simulink model "Position_Control_PID_CSEI"  (R2023b)
settings: Solver=FixedStepAuto  StartTime=0.0  StopTime=T_final  FixedStep=0.01  RelTol=1e-3
values from neighbouring files (symbols this model uses):
  current = [0;0]    [ASMC_ESO_sim_CSEI_Scripts.m]    (also in ASMC_FTESO_sim_CSEI_Scripts.m; Berthing_Control_PID_CSEI_Scripts.m; Position_Control_PID_CSEI_Scripts.m; Position_Control_PID_CSEI_Scripts_released.m)
  f_BT_max = 0.3*10    (= 3)    [Berthing_Control_PID_CSEI_Scripts.m]    (also in Control_allocation_test.m = 0.3; Position_Control_PID_CSEI_Scripts.m; Position_Control_PID_CSEI_Scripts_released.m; Waypoint_Control_PID_CSEI_Scripts.m)
  f_VSP1_max = 0.45*10    (= 4.5)    [Berthing_Control_PID_CSEI_Scripts.m]    (also in Control_allocation_test.m = 0.45; Position_Control_PID_CSEI_Scripts.m; Position_Control_PID_CSEI_Scripts_released.m; Waypoint_Control_PID_CSEI_Scripts.m)
  f_VSP2_max = 0.45*10    (= 4.5)    [Berthing_Control_PID_CSEI_Scripts.m]    (also in Control_allocation_test.m = 0.45; Position_Control_PID_CSEI_Scripts.m; Position_Control_PID_CSEI_Scripts_released.m; Waypoint_Control_PID_CSEI_Scripts.m)
  Fx_max = f_VSP1_max + f_VSP2_max    (= 9)    [Berthing_Control_PID_CSEI_Scripts.m]    (also in Control_allocation_test.m = 0.9; Position_Control_PID_CSEI_Scripts.m; Position_Control_PID_CSEI_Scripts_released.m; Waypoint_Control_PID_CSEI_Scripts.m)
  Fx_min = 0    [Berthing_Control_PID_CSEI_Scripts.m]    (also in Control_allocation_test.m = -0.9; Position_Control_PID_CSEI_Scripts.m; Position_Control_PID_CSEI_Scripts_released.m = -9; Waypoint_Control_PID_CSEI_Scripts.m)
  Fy_max = f_VSP1_max + f_VSP2_max + f_BT_max    (= 12)    [Berthing_Control_PID_CSEI_Scripts.m]    (also in Control_allocation_test.m = 1.2; Position_Control_PID_CSEI_Scripts.m; Position_Control_PID_CSEI_Scripts_released.m; Waypoint_Control_PID_CSEI_Scripts.m)
  Fy_min = -Fy_max    (= -12)    [Berthing_Control_PID_CSEI_Scripts.m]    (also in Control_allocation_test.m = -1.2; Position_Control_PID_CSEI_Scripts.m; Position_Control_PID_CSEI_Scripts_released.m; Waypoint_Control_PID_CSEI_Scripts.m)
  Kanti_u = 0.02    [Berthing_Control_PID_CSEI_Scripts.m]    (also in Position_Control_PID_CSEI_Scripts.m = 0; Waypoint_Control_PID_CSEI_Scripts.m; Waypoint_Control_PID_CSEI_Scripts_LLA.m)
  Kanti_x = 0    [Position_Control_PID_CSEI_Scripts.m]
  Kanti_y = 0    [Position_Control_PID_CSEI_Scripts.m]
  Kd_psi = 10    [Berthing_Control_PID_CSEI_Scripts.m]    (also in Position_Control_PID_CSEI_Scripts.m = 30; Waypoint_Control_PID_CSEI_Scripts.m; Waypoint_Control_PID_CSEI_Scripts_LLA.m)
  Kd_u = 1    [Berthing_Control_PID_CSEI_Scripts.m]    (also in Position_Control_PID_CSEI_Scripts.m = 7; Waypoint_Control_PID_CSEI_Scripts.m; Waypoint_Control_PID_CSEI_Scripts_LLA.m)
  Kd_v = 0    [Position_Control_PID_CSEI_Scripts.m]
  Kd_x = 0    [Position_Control_PID_CSEI_Scripts.m]
  Kd_y = 5    [Position_Control_PID_CSEI_Scripts.m]
  Ki_u = 2    [Berthing_Control_PID_CSEI_Scripts.m]    (also in Position_Control_PID_CSEI_Scripts.m = 0; Waypoint_Control_PID_CSEI_Scripts.m; Waypoint_Control_PID_CSEI_Scripts_LLA.m)
  Ki_x = 0    [Position_Control_PID_CSEI_Scripts.m]
  Ki_y = 0    [Position_Control_PID_CSEI_Scripts.m]
  Kp_psi = 100    [Berthing_Control_PID_CSEI_Scripts.m]    (also in Position_Control_PID_CSEI_Scripts.m = 50; Waypoint_Control_PID_CSEI_Scripts.m; Waypoint_Control_PID_CSEI_Scripts_LLA.m)
  Kp_u = 21    [Berthing_Control_PID_CSEI_Scripts.m]    (also in Position_Control_PID_CSEI_Scripts.m = 1; Waypoint_Control_PID_CSEI_Scripts.m; Waypoint_Control_PID_CSEI_Scripts_LLA.m)
  Kp_v = 1.2    [Position_Control_PID_CSEI_Scripts.m]
  Kp_x = 0.7    [Position_Control_PID_CSEI_Scripts.m]
  Kp_y = 0.3    [Position_Control_PID_CSEI_Scripts.m]
  N_max = Fx_max*ly_VSP*(1) - Fx_max*ly_VSP*(-1) + f_BT_max*lx_BT    (= 2.1525)    [Berthing_Control_PID_CSEI_Scripts.m]    (also in Control_allocation_test.m = 0.16575; Position_Control_PID_CSEI_Scripts.m; Position_Control_PID_CSEI_Scripts_released.m; Waypoint_Control_PID_CSEI_Scripts.m)
  N_min = -N_max    (= -2.1525)    [Berthing_Control_PID_CSEI_Scripts.m]    (also in Control_allocation_test.m = -0.16575; Position_Control_PID_CSEI_Scripts.m; Position_Control_PID_CSEI_Scripts_released.m; Waypoint_Control_PID_CSEI_Scripts.m)
  Nu = 100    [Position_Control_PID_CSEI_Scripts.m]
  Nv = 100    [Position_Control_PID_CSEI_Scripts.m]
  Nx = 100    [Position_Control_PID_CSEI_Scripts.m]
  Ny = 100    [Position_Control_PID_CSEI_Scripts.m]
  psi_ref_deg = 50    [Position_Control_PID_CSEI_Scripts.m]    (also in Position_Control_PID_CSEI_Scripts_released.m = 30)
  u_max = 2    [Position_Control_PID_CSEI_Scripts.m]    (also in Position_Control_PID_CSEI_Scripts_released.m)
  u_min = -2    [Position_Control_PID_CSEI_Scripts.m]    (also in Position_Control_PID_CSEI_Scripts_released.m)
  u_vsp_min = 0    [Position_Control_PID_CSEI_Scripts.m]    (also in Position_Control_PID_CSEI_Scripts_released.m)
  v_max = 10    [ASMC_ESO_sim_CSEI_Scripts.m]    (also in ASMC_FTESO_sim_CSEI_Scripts.m; Position_Control_PID_CSEI_Scripts.m = 2; Position_Control_PID_CSEI_Scripts_released.m = 2; SMC_ESO_sim_CSEI_Scripts.m)
  v_min = -v_max    (= -0.25)    [ASMC_ESO_sim_CSEI_Scripts.m]    (also in ASMC_FTESO_sim_CSEI_Scripts.m; Position_Control_PID_CSEI_Scripts.m = -2; Position_Control_PID_CSEI_Scripts_released.m = -2; SMC_ESO_sim_CSEI_Scripts.m)
  x0 = zeros(6,1)    [Berthing_Control_PID_CSEI_Scripts.m]    (also in Position_Control_PID_CSEI_Scripts.m; Position_Control_PID_CSEI_Scripts_released.m; Waypoint_Control_PID_CSEI_Scripts.m; Waypoint_Control_PID_CSEI_Scripts_LLA.m)
  x_dock = 20    [Position_Control_PID_CSEI_Scripts.m]    (also in Position_Control_PID_CSEI_Scripts_released.m = 30)
  y_dock = 20    [Position_Control_PID_CSEI_Scripts.m]    (also in Position_Control_PID_CSEI_Scripts_released.m = 30)
libraries: simulink_extras x4, vrlib x2
settings Model: Creator=ADMIN  LastModifiedBy=ADMIN
settings ModelReferenceCC: EnableRefExpFcnMdlSchedulingChecks=on

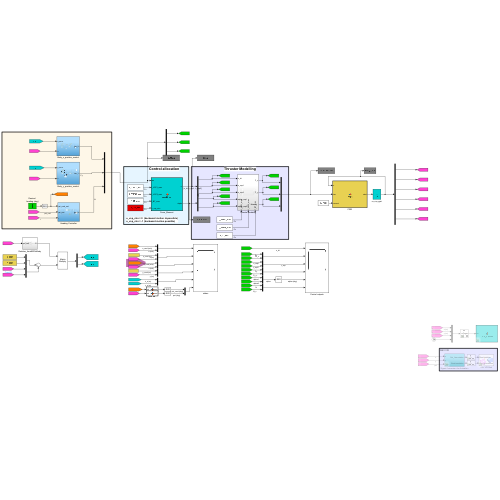
[thumbnail: Simulink's stored preview of the top-level diagram]
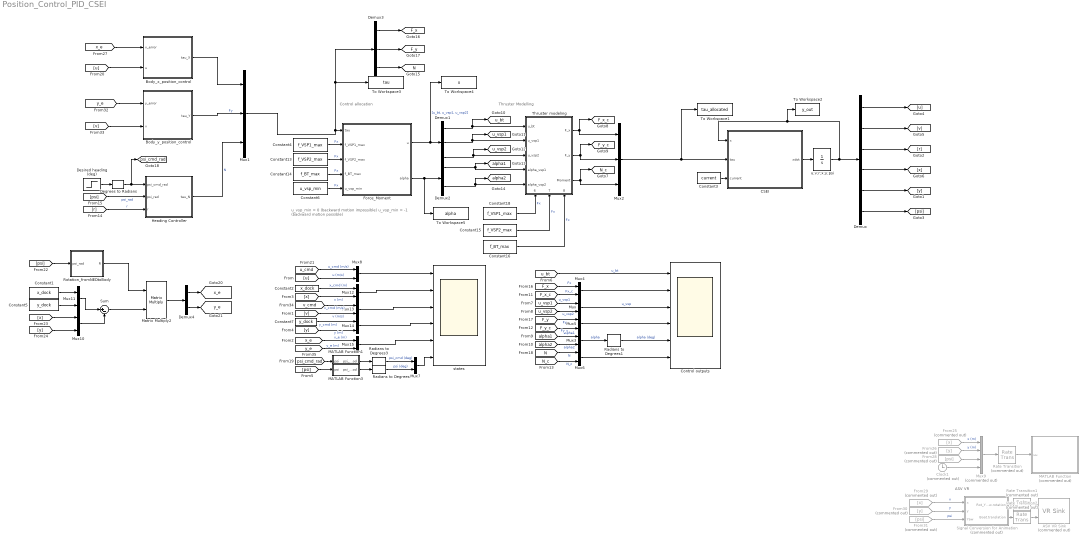
== system Position_Control_PID_CSEI ==
  note: u_vsp_min = 0 (backward motion impossible)
      | u_vsp_min = -1 (backward motion possible)
  note: Thruster Modelling
  note: ASV VR
  note: Control allocation
  ASV VR Sink : vrlib/VR Sink  Commented=on  InstantiateOnLoad=on  SampleTime=0.1  ViewEnable=on  RemoteChange=off  RemoteView=off  FieldsWritten=Boat.rotation.4.1.1.double#Boat.translation.3.1.1.double  WorldFileName=ASV.x3d  WorldDescription=ASV Simulation Animation  AutoView=off  VideoDimensions=[]  AllowVariableSize=off
  Body_x_position_control : Subsystem
  Body_y_position_control : Subsystem
  CSEI : MATLAB Function  TreatAsAtomicUnit=on
  Clock1 : Clock  Commented=on
  Constant1 : Constant  Value=x_dock
  Constant13 : Constant  Value=f_VSP2_max
  Constant14 : Constant  Value=f_BT_max
  Constant15 : Constant  Value=f_VSP2_max
  Constant16 : Constant  Value=f_BT_max
  Constant18 : Constant  Value=f_VSP1_max
  Constant2 : Constant  Value=x_dock
  Constant3 : Constant  Value=current
  Constant4 : Constant  Value=f_VSP1_max
  Constant5 : Constant  Value=y_dock
  Constant6 : Constant  Value=u_vsp_min
  Constant7 : Constant  Value=y_dock
  Control outputs : Scope  NumInputPorts=6
  Degrees to Radians : simulink_extras/Transformations/Degrees to Radians
  Demux : Demux  Outputs=6
  Demux1 : Demux  Outputs=3
  Demux2 : Demux  Outputs=2
  Demux3 : Demux  Outputs=3
  Demux4 : Demux  Outputs=2
  Desired heading (deg) : Step  Time=0  After=psi_ref_deg  SampleTime=0
  Force_Moment : MATLAB Function  TreatAsAtomicUnit=on
  From25 : From  Commented=on  GotoTag=x
  From26 : From  Commented=on  GotoTag=y
  From28 : From  Commented=on  GotoTag=psi
  From29 : From  Commented=on  GotoTag=x
  From30 : From  Commented=on  GotoTag=y
  From31 : From  Commented=on  GotoTag=psi
  Heading Controller : Subsystem
  MATLAB Function : MATLAB Function  Commented=on  TreatAsAtomicUnit=on
  MATLAB Function1 : MATLAB Function  TreatAsAtomicUnit=on
  MATLAB Function3 : MATLAB Function  TreatAsAtomicUnit=on
  Matrix Multiply2 : Product  Multiplication=Matrix(*)
  Mux{,3..8,10..15} (13 alike) : Mux  Inputs=2
  Mux1 : Mux  Inputs=3
  Mux2 : Mux  Inputs=3
  Mux9 : Mux  Commented=on
  Radians to Degrees : simulink_extras/Transformations/Radians to Degrees
  Radians to Degrees1 : simulink_extras/Transformations/Radians to Degrees
  Radians to Degrees3 : simulink_extras/Transformations/Radians to Degrees
  Rate Transition : RateTransition  Commented=on  OutPortSampleTime=5
  Rate Transition1 : RateTransition  Commented=on  OutPortSampleTime=5
  Rate Transition2 : RateTransition  Commented=on  OutPortSampleTime=5
  Rotation_fromNEDtoBody : Subsystem
  Signal Conversion for Animation : Subsystem  Commented=on
  Sum : Sum  Inputs=|+-
  Thruster modeling : Subsystem
      settings: PortSchema="{\"entries\":[{\"content\":{\"sides\":[{\"content\":{\"connectorIds\":[\"In1\",\"In2\",\"In3\",\"In4\",\"In5\"]},\"type\":\"ConnectorPlacement.EquallySpacedRectSide\",\"uuid\":\"a022356d-9f83-420f-8db1-af87d581b43a\"},{\"content\":{\"connectorIds\":[\"Out1\",\"Out2\",\"Out3\"],\"side\":\"RIGHT\"},\"type\":\"ConnectorPlacement.EquallySpacedRectSide\",\"uuid\":\"80059f0e-998a-4ca1-ad21-b5517d0d415e\"},{\"content\":{\"side\":\"TOP\"},\"type\":\"ConnectorPlacement.EquallySpacedRectSide\",\"uuid\":\"bbd861b1-62fd-403d-9398-039fcb3ecf9c\"},{\"content\":{\"connectorIds\":[\"In6\",\"In7\",\"In8\"],\"side\":\"BOTTOM\"},\"type\":\"ConnectorPlacement.EquallySpacedRectSide\",\"uuid\":\"ab01237b-8b46-48b2-b107-c489b1f78e8c\"}]},\"type\":\"ConnectorPlacement.EquallySpacedConnector\",\"uuid\":\"7da2a0ce-fa7c-4136-9950-942e5a1638e8\"}],\"packageUris\":[\"http://schema.mathworks.com/mf0/Connector/R2020b\"],\"version\":\"1.0\"}"
  To Workspace1 : ToWorkspace  VariableName=tau_allocated  SampleTime=-1
  To Workspace2 : ToWorkspace  VariableName=y_out  SampleTime=-1
  To Workspace3 : ToWorkspace  VariableName=tau  SampleTime=-1
  To Workspace4 : ToWorkspace  VariableName=u  SampleTime=-1
  To Workspace5 : ToWorkspace  VariableName=alpha  SampleTime=-1
  states : Scope  NumInputPorts=6
  u;v;r;x;y;psi : Integrator  InitialCondition=x0
  tag scope: F_x=global, F_x_c=global, F_y=global, F_y_c=global, N=global, N_c=global, alpha1=global, alpha2=global, psi_cmd_rad=global, u_bt=global, u_vsp1=global, u_vsp2=global, x_e=global, y_e=global
  wires:
  Mux2/1 -> To Workspace1/1, CSEI/2(tau)
  CSEI/1(xdot) -> u;v;r;x;y;psi/1
  u;v;r;x;y;psi/1 -> Demux/1, To Workspace2/1, CSEI/1(x)
  Constant3/1 -> CSEI/3(current)
  Thruster modeling/1(F_x) -> Mux2/1, [F_x_c]
  Thruster modeling/2(F_y) -> Mux2/2, [F_y_c]
  Thruster modeling/3("Moment ") -> Mux2/3, [N_c]
  Demux/6 -> [psi]
  Demux/1 -> [u]
  Demux/4 -> [x]
  Demux/5 -> [y]
  Demux/3 -> [r]
  Demux/2 -> [v]
  Demux2/1 -> Thruster modeling/4(alpha_vsp1), [alpha1]
  Demux1/2 -> Thruster modeling/2(u_vsp1), [u_vsp1]
  Demux1/1 -> Thruster modeling/1(u_bt), [u_bt]
  [u_vsp1] -> Mux/1  "u_vsp1"
  [u_vsp2] -> Mux/2  "u_vsp2"
  [alpha1] -> Mux3/1  "alpha1"
  [alpha2] -> Mux3/2  "alpha2"
  [u_bt] -> Control outputs/1  "u_bt"
  Mux/1 -> Control outputs/3  "u_vsp"
  [F_x_c] -> Mux4/2  "Fx_c"
  Mux3/1 -> Radians to Degrees1/1  "alpha"
  Radians to Degrees1/1 -> Control outputs/5  "alpha (deg)"
  Demux2/2 -> [alpha2], Thruster modeling/5(alpha_vsp2)
  Demux1/3 -> [u_vsp2], Thruster modeling/3("u_vsp2 ")
  Force_Moment/1(u) -> To Workspace4/1, Demux1/1  "[u_bt, u_vsp1, u_vsp2]"
  Force_Moment/2(alpha) -> To Workspace5/1, Demux2/1
  [psi] -> Heading Controller/2(psi_rad)  "psi_rad"
  [r] -> Heading Controller/3(r)  "r"
  Heading Controller/1(tau_N) -> Mux1/3  "N"
  Body_y_position_control/1(tau_Y) -> Mux1/2  "Fy"
  [F_x] -> Mux4/1  "Fx"
  Mux4/1 -> Control outputs/2
  [F_y] -> Mux5/1  "Fy"
  [F_y_c] -> Mux5/2  "Fy_c"
  Mux5/1 -> Control outputs/4
  [N] -> Mux6/1  "N"
  [N_c] -> Mux6/2  "N_c"
  Mux6/1 -> Control outputs/6
  Constant4/1 -> Force_Moment/2(f_VSP1_max)  "Fx"
  [u] -> Body_x_position_control/2(u)
  Body_x_position_control/1(tau_X) -> Mux1/1
  Clock1/1 -> Mux9/4
  From26/1 -> Mux9/2  "y (m)"
  From25/1 -> Mux9/1  "x (m)"
  Mux9/1 -> Rate Transition/1
  From28/1 -> Mux9/3
  Rate Transition/1 -> MATLAB Function/1(uu)
  Signal Conversion for Animation/1(Rot_Yaw.rotation) -> Rate Transition1/1
  Signal Conversion for Animation/2(Boat.translation) -> Rate Transition2/1
  From30/1 -> Signal Conversion for Animation/2(y)  "y"
  From31/1 -> Signal Conversion for Animation/3(Yaw)  "psi"
  From29/1 -> Signal Conversion for Animation/1(x)  "x"
  Rate Transition1/1 -> ASV VR Sink/1
  Rate Transition2/1 -> ASV VR Sink/2
  Degrees to Radians/1 -> [psi_cmd_rad], Heading Controller/1(psi_cmd_rad)
  Mux1/1 -> Demux3/1, To Workspace3/1, Force_Moment/1(tau)
  Demux3/1 -> [F_x]
  Demux3/2 -> [F_y]
  Demux3/3 -> [N]
  Constant13/1 -> Force_Moment/3(f_VSP2_max)  "Fx"
  Constant14/1 -> Force_Moment/4(f_BT_max)  "Fx"
  Constant18/1 -> Thruster modeling/6(f_VSP1_max)  "Fx"
  Constant15/1 -> Thruster modeling/7(f_VSP2_max)  "Fx"
  Constant16/1 -> Thruster modeling/8(f_BT_max)  "Fx"
  Desired heading (deg)/1 -> Degrees to Radians/1
  [psi] -> Rotation_fromNEDtoBody/1(psi_rad)
  Demux4/2 -> [y_e]
  Rotation_fromNEDtoBody/1(R) -> Matrix Multiply2/1
  Matrix Multiply2/1 -> Demux4/1
  Demux4/1 -> [x_e]
  [x] -> Mux10/1
  Sum/1 -> Matrix Multiply2/2
  [y] -> Mux10/2
  Constant5/1 -> Mux11/2
  Constant1/1 -> Mux11/1
  Mux11/1 -> Sum/1
  Mux10/1 -> Sum/2
  [x_e] -> Body_x_position_control/1(x_error)
  [y_e] -> Body_y_position_control/1(y_error)
  [v] -> Body_y_position_control/2(v)
  Constant2/1 -> Mux12/1  "x_cmd (m)"
  Radians to Degrees3/1 -> Mux7/1  "psi_cmd (deg)"
  [v] -> Mux13/2  "v (m/s)"
  [psi_cmd_rad] -> MATLAB Function1/1(psi)
  Mux8/1 -> states/1
  Mux15/1 -> states/5
  [u_cmd] -> Mux8/1  "u_cmd (m/s)"
  Mux7/1 -> states/6
  MATLAB Function1/1(psi_mod) -> Radians to Degrees3/1
  [psi] -> MATLAB Function3/1(psi)
  [x] -> Mux12/2  "x (m)"
  [y] -> Mux14/2  "y (m)"
  Mux12/1 -> states/2
  Radians to Degrees/1 -> Mux7/2  "psi (deg)"
  MATLAB Function3/1(psi_mod) -> Radians to Degrees/1
  [u] -> Mux8/2  "u (m/s)"
  Mux13/1 -> states/3
  [v_cmd] -> Mux13/1  "v_cmd (m/s)"
  Mux14/1 -> states/4
  Constant7/1 -> Mux14/1  "y_cmd (m)"
  [x_e] -> Mux15/1  "x_e (m)"
  [y_e] -> Mux15/2  "y_e (m)"
  Constant6/1 -> Force_Moment/5(u_vsp_min)  "Fx"

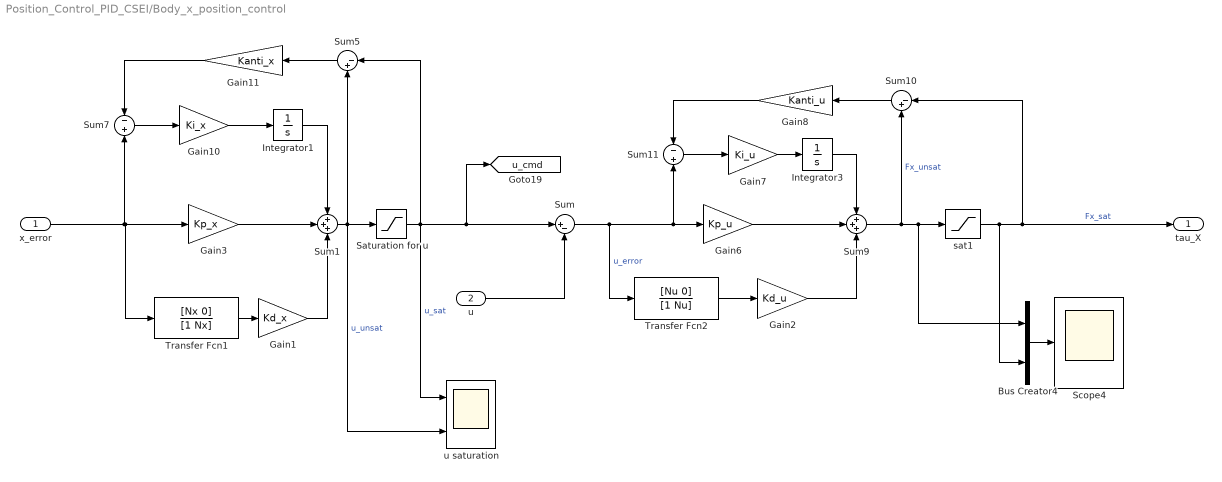
== system Position_Control_PID_CSEI/Body_x_position_control ==
  x_error : Inport
  u : Inport  Port=2
  Bus Creator4 : BusCreator  Inputs=2
  Gain1 : Gain  Gain=Kd_x
  Gain10 : Gain  Gain=Ki_x
  Gain11 : Gain  Gain=Kanti_x
  Gain2 : Gain  Gain=Kd_u
  Gain3 : Gain  Gain=Kp_x
  Gain6 : Gain  Gain=Kp_u
  Gain7 : Gain  Gain=Ki_u
  Gain8 : Gain  Gain=Kanti_u
  Integrator1 : Integrator
  Integrator3 : Integrator
  Saturation for u : Saturate  UpperLimit=u_max  LowerLimit=u_min
  Scope4 : Scope
  Sum : Sum  Inputs=|+-
  Sum1 : Sum  Inputs=+++  InputSameDT=on  SaturateOnIntegerOverflow=on  OutDataTypeStr=Inherit: Same as first input
  Sum10 : Sum  Inputs=|-+  InputSameDT=on  SaturateOnIntegerOverflow=on  OutDataTypeStr=Inherit: Same as first input
  Sum11 : Sum  Inputs=-|+  InputSameDT=on  SaturateOnIntegerOverflow=on  OutDataTypeStr=Inherit: Same as first input
  Sum5 : Sum  Inputs=|-+  InputSameDT=on  SaturateOnIntegerOverflow=on  OutDataTypeStr=Inherit: Same as first input
  Sum7 : Sum  Inputs=-|+  InputSameDT=on  SaturateOnIntegerOverflow=on  OutDataTypeStr=Inherit: Same as first input
  Sum9 : Sum  Inputs=+++  InputSameDT=on  SaturateOnIntegerOverflow=on  OutDataTypeStr=Inherit: Same as first input
  Transfer Fcn1 : TransferFcn  Numerator=[Nx 0]  Denominator=[1 Nx]
  Transfer Fcn2 : TransferFcn  Numerator=[Nu 0]  Denominator=[1 Nu]
  sat1 : Saturate  UpperLimit=Fx_max  LowerLimit=Fx_min
      settings: AttributesFormatString=%<LowerLimit>~%<UpperLimit>
  u saturation : Scope  NumInputPorts=2
  tau_X : Outport
  tag scope: u_cmd=global
  wires:
  Gain7/1 -> Integrator3/1
  Sum/1 -> Transfer Fcn2/1, Gain6/1, Sum11/2  "u_error"
  sat1/1 -> tau_X/1, Sum10/1, Bus Creator4/2  "Fx_sat"
  Bus Creator4/1 -> Scope4/1
  Transfer Fcn2/1 -> Gain2/1
  Sum9/1 -> Bus Creator4/1, sat1/1, Sum10/2  "Fx_unsat"
  Sum10/1 -> Gain8/1
  Integrator3/1 -> Sum9/1
  Gain2/1 -> Sum9/3
  Gain8/1 -> Sum11/1
  Gain6/1 -> Sum9/2
  Sum11/1 -> Gain7/1
  u/1 -> Sum/2
  Sum5/1 -> Gain11/1
  Saturation for u/1 -> [u_cmd], Sum/1, u saturation/1, Sum5/1  "u_sat"
  Sum7/1 -> Gain10/1
  Gain3/1 -> Sum1/2
  Gain11/1 -> Sum7/1
  Integrator1/1 -> Sum1/1
  Gain1/1 -> Sum1/3
  Sum1/1 -> u saturation/2, Sum5/2, Saturation for u/1  "u_unsat"
  Gain10/1 -> Integrator1/1
  x_error/1 -> Transfer Fcn1/1, Gain3/1, Sum7/2
  Transfer Fcn1/1 -> Gain1/1

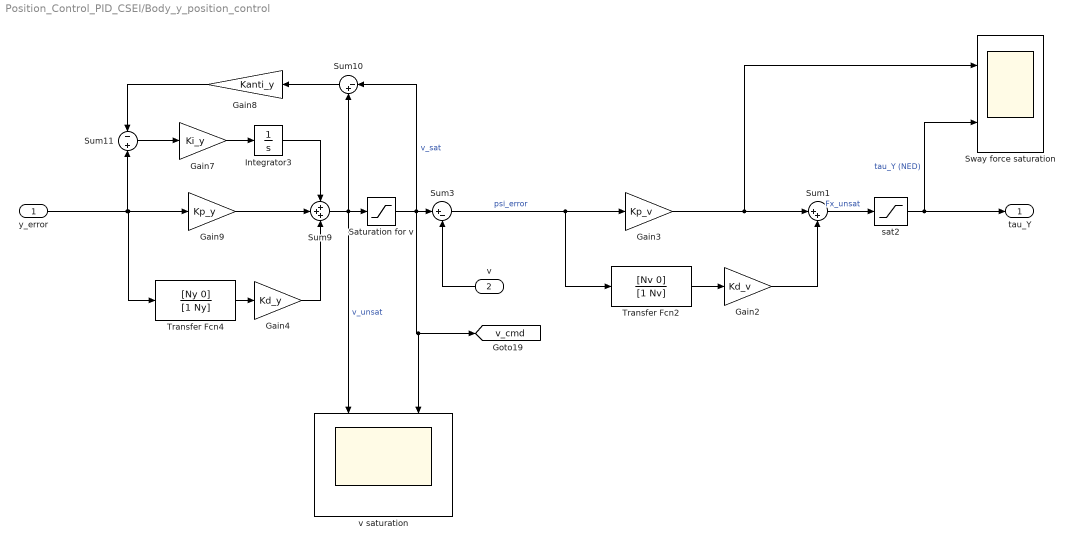
== system Position_Control_PID_CSEI/Body_y_position_control ==
  y_error : Inport
  v : Inport  Port=2
  Gain2 : Gain  Gain=Kd_v
  Gain3 : Gain  Gain=Kp_v
  Gain4 : Gain  Gain=Kd_y
  Gain7 : Gain  Gain=Ki_y
  Gain8 : Gain  Gain=Kanti_y
  Gain9 : Gain  Gain=Kp_y
  Integrator3 : Integrator
  Saturation for v : Saturate  UpperLimit=v_max  LowerLimit=v_min
  Sum1 : Sum  Inputs=|++  InputSameDT=on  SaturateOnIntegerOverflow=on  OutDataTypeStr=Inherit: Same as first input
  Sum10 : Sum  Inputs=|-+  InputSameDT=on  SaturateOnIntegerOverflow=on  OutDataTypeStr=Inherit: Same as first input
  Sum11 : Sum  Inputs=-|+  InputSameDT=on  SaturateOnIntegerOverflow=on  OutDataTypeStr=Inherit: Same as first input
  Sum3 : Sum  Inputs=|+-  InputSameDT=on  SaturateOnIntegerOverflow=on  OutDataTypeStr=Inherit: Same as first input
  Sum9 : Sum  Inputs=+++  InputSameDT=on  SaturateOnIntegerOverflow=on  OutDataTypeStr=Inherit: Same as first input
  Sway force saturation : Scope  NumInputPorts=2
  Transfer Fcn2 : TransferFcn  Numerator=[Nv 0]  Denominator=[1 Nv]
  Transfer Fcn4 : TransferFcn  Numerator=[Ny 0]  Denominator=[1 Ny]
  sat2 : Saturate  UpperLimit=Fy_max  LowerLimit=Fy_min
      settings: AttributesFormatString=%<LowerLimit>~%<UpperLimit>
  v saturation : Scope  NumInputPorts=2
  tau_Y : Outport
  tag scope: v_cmd=global
  wires:
  Sum10/1 -> Gain8/1
  y_error/1 -> Sum11/2, Gain9/1, Transfer Fcn4/1
  Gain3/1 -> Sum1/1, Sway force saturation/1
  sat2/1 -> Sway force saturation/2, tau_Y/1  "tau_Y (NED)"
  Gain9/1 -> Sum9/2
  Saturation for v/1 -> [v_cmd], v saturation/2, Sum10/1, Sum3/1  "v_sat"
  Gain7/1 -> Integrator3/1
  Sum11/1 -> Gain7/1
  Integrator3/1 -> Sum9/1
  Gain8/1 -> Sum11/1
  Sum9/1 -> v saturation/1, Sum10/2, Saturation for v/1  "v_unsat"
  Transfer Fcn4/1 -> Gain4/1
  Gain4/1 -> Sum9/3
  Sum3/1 -> Transfer Fcn2/1, Gain3/1  "psi_error"
  v/1 -> Sum3/2
  Transfer Fcn2/1 -> Gain2/1
  Gain2/1 -> Sum1/2
  Sum1/1 -> sat2/1  "Fx_unsat"

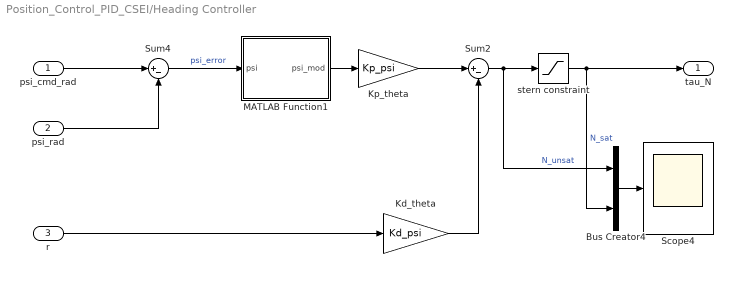
== system Position_Control_PID_CSEI/Heading Controller ==
  psi_cmd_rad : Inport
  psi_rad : Inport  Port=2
  r : Inport  Port=3
  Bus Creator4 : BusCreator  Inputs=2
  Kd_theta : Gain  Gain=Kd_psi  SaturateOnIntegerOverflow=on  OutDataTypeStr=Inherit: Same as input  ParamDataTypeStr=Inherit: Same as input
  Kp_theta : Gain  Gain=Kp_psi  SaturateOnIntegerOverflow=on  OutDataTypeStr=Inherit: Same as input  ParamDataTypeStr=Inherit: Same as input
  MATLAB Function1 : MATLAB Function  TreatAsAtomicUnit=on
  Scope4 : Scope
  Sum2 : Sum  Inputs=|+-  InputSameDT=on  SaturateOnIntegerOverflow=on  OutDataTypeStr=Inherit: Same as first input
  Sum4 : Sum  Inputs=|+-  InputSameDT=on  SaturateOnIntegerOverflow=on  OutDataTypeStr=Inherit: Same as first input
  stern constraint : Saturate  UpperLimit=N_max  LowerLimit=N_min
      settings: AttributesFormatString=%<LowerLimit>~%<UpperLimit>
  tau_N : Outport
  wires:
  Kp_theta/1 -> Sum2/1
  MATLAB Function1/1(psi_mod) -> Kp_theta/1
  psi_cmd_rad/1 -> Sum4/1
  Sum4/1 -> MATLAB Function1/1(psi)  "psi_error"
  Kd_theta/1 -> Sum2/2
  r/1 -> Kd_theta/1
  psi_rad/1 -> Sum4/2
  Sum2/1 -> Bus Creator4/1, stern constraint/1  "N_unsat"
  Bus Creator4/1 -> Scope4/1
  stern constraint/1 -> Bus Creator4/2, tau_N/1  "N_sat"

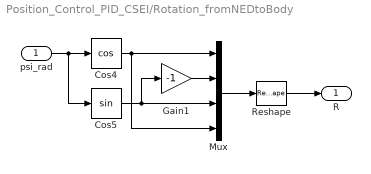
== system Position_Control_PID_CSEI/Rotation_fromNEDtoBody ==
  psi_rad : Inport
  Cos4 : Trigonometry  Operator=cos
  Cos5 : Trigonometry
  Gain1 : Gain  Gain=-1
  Mux : Mux
  Reshape : Reshape  OutputDimensionality=Customize  OutputDimensions=[2,2]
  R : Outport
  wires:
  psi_rad/1 -> Cos5/1, Cos4/1
  Mux/1 -> Reshape/1
  Cos4/1 -> Mux/1, Mux/4
  Cos5/1 -> Mux/3, Gain1/1
  Reshape/1 -> R/1
  Gain1/1 -> Mux/2

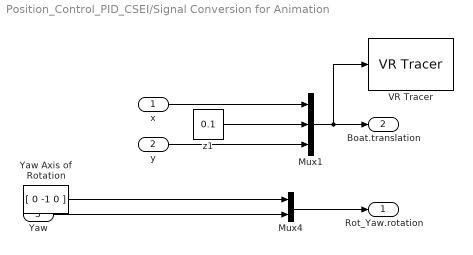
== system Position_Control_PID_CSEI/Signal Conversion for Animation ==
  x : Inport
  y : Inport  Port=2
  Yaw : Inport  Port=3
  Mux1 : Mux  Inputs=3
  Mux4 : Mux  Inputs=2
  VR Tracer : vrlib/VR Tracer  VrmlFile=ASV.x3d  MarkerName=None  UseLines=on  UseTriads=off  MarkerScale=[1 1 1]  MarkerColorSelection=Defined as RGB values  MarkerColor=red  rgbval=[1 0 0]  Ts=0.5  ForceViewerOpen=off  ConnectPlane=off  PlaneCoeff=[0 1 0 0]  ConnectPoint=None  PointCoord=[0 0 0]
  Yaw Axis of Rotation : Constant  Value=[ 0 -1 0 ]
  z1 : Constant  Value=0.1
  Rot_Yaw.rotation : Outport
  Boat.translation : Outport  Port=2
  wires:
  Yaw Axis of Rotation/1 -> Mux4/1
  Mux1/1 -> VR Tracer/1, Boat.translation/1
  x/1 -> Mux1/1
  Mux4/1 -> Rot_Yaw.rotation/1
  Yaw/1 -> Mux4/2
  y/1 -> Mux1/3
  z1/1 -> Mux1/2

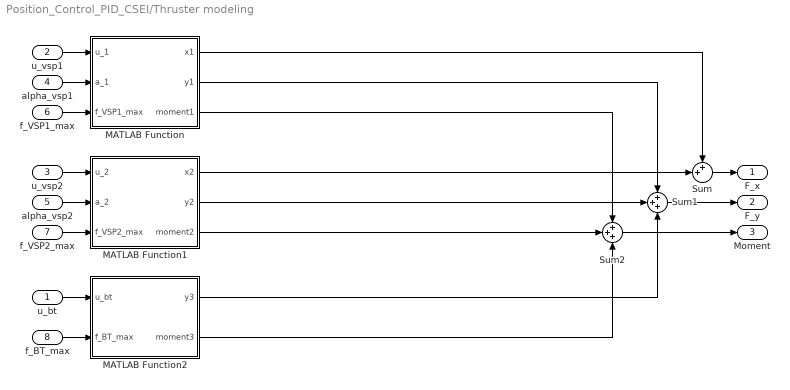
== system Position_Control_PID_CSEI/Thruster modeling ==
  u_bt : Inport
  u_vsp1 : Inport  Port=2
  "u_vsp2 " : Inport  Port=3
  alpha_vsp1 : Inport  Port=4
  alpha_vsp2 : Inport  Port=5
  f_VSP1_max : Inport  Port=6
  f_VSP2_max : Inport  Port=7
  f_BT_max : Inport  Port=8
  MATLAB Function : MATLAB Function  TreatAsAtomicUnit=on
  MATLAB Function1 : MATLAB Function  TreatAsAtomicUnit=on
  MATLAB Function2 : MATLAB Function  TreatAsAtomicUnit=on
  Sum : Sum  Inputs=++|
  Sum1 : Sum  Inputs=+++
  Sum2 : Sum  Inputs=+++
  F_x : Outport
  F_y : Outport  Port=2
  "Moment " : Outport  Port=3
  wires:
  u_bt/1 -> MATLAB Function2/1(u_bt)
  alpha_vsp2/1 -> MATLAB Function1/2(a_2)
  u_vsp1/1 -> MATLAB Function/1(u_1)
  "u_vsp2 "/1 -> MATLAB Function1/1(u_2)
  MATLAB Function1/1(x2) -> Sum/2
  Sum/1 -> F_x/1
  Sum1/1 -> F_y/1
  MATLAB Function1/2(y2) -> Sum1/2
  MATLAB Function2/1(y3) -> Sum1/3
  Sum2/1 -> "Moment "/1
  MATLAB Function2/2(moment3) -> Sum2/3
  MATLAB Function1/3(moment2) -> Sum2/2
  MATLAB Function/3(moment1) -> Sum2/1
  MATLAB Function/1(x1) -> Sum/1
  MATLAB Function/2(y1) -> Sum1/1
  alpha_vsp1/1 -> MATLAB Function/2(a_1)
  f_VSP1_max/1 -> MATLAB Function/3(f_VSP1_max)
  f_VSP2_max/1 -> MATLAB Function1/3(f_VSP2_max)
  f_BT_max/1 -> MATLAB Function2/2(f_BT_max)

== matlab function Position_Control_PID_CSEI/Force_Moment ==
  data: tau input; u output; alpha output; f_VSP1_max input; f_VSP2_max input; f_BT_max input; u_vsp_min input
function [u, alpha] = force2input(tau, f_VSP1_max, f_VSP2_max, f_BT_max, u_vsp_min)
    % Mapping of desired force (tau) to input to the actuators (u)
    % Input: 3DOF desired forces and moment in body-frame, tau = [X Y N]'
    % Output: input signals to the actuators, u = [u_BT u_VSP1 u_VSP2]';
    %         angles of the two VSPs, alpha = [alpha_VSP1 alpha_VSP2]';
    %         angular rates of the VSPs, omega = [omega_VSP1 omega_VSP2]'
%% Initializing values
    ly_VSP = 0.055;         % Moment arm along y for VSP
    lx_VSP = 0.4574;        % Moment arm along x for VSP
    lx_BT = 0.3875;         % Moment arm along x for BT

    % test
    alpha = zeros(2,1);     % VSP angles
    u = zeros(3,1);         % Input vector to the VSPs and BT

    B = [  1      0       1      0      0;
           0      1       0      1      1;
         ly_VSP -lx_VSP -ly_VSP -lx_VSP lx_BT]; % Configuration matrix
%% Thrust allocation
    B_inv = pinv(B);                         % Calculating dagger
    f_cmd = B_inv*tau;                       % Forces and moment

    u_cmd = [norm(f_cmd(1:2))/f_VSP1_max;
             norm(f_cmd(3:4))/f_VSP2_max;
             f_cmd(5)/f_BT_max];                % Calculating input to each
                                                % thruster
    % Saturation: Limit input signal to VSPs to be within [0,1]
    if u_cmd(1) < u_vsp_min
        u_cmd(1) = u_vsp_min;
    elseif u_cmd(1) > 1
        u_cmd(1) = 1;
    else
        u_cmd(1) = u_cmd(1);
    end

    if u_cmd(2) < u_vsp_min
        u_cmd(2) = u_vsp_min;
    elseif u_cmd(2) > 1
        u_cmd(2) = 1;
    else
        u_cmd(2) = u_cmd(2);
    end

    % Saturation: Limit input signal to BT to be within [-1,1]
    if u_cmd(3) < -1
        u_cmd(3) = -1;
    elseif u_cmd(3) > 1
        u_cmd(3) = 1;
    else
        u_cmd(3) = u_cmd(3);
    end
    
    alpha(1) = atan2(f_cmd(2),f_cmd(1));         % Calculate angle of VSP1
    alpha(2) = atan2(f_cmd(4),f_cmd(3));         % Calculate angle of VSP2
    BT_gain = 1;                                 % Gain used in LAB

    u(1) = u_cmd(3)*BT_gain;                     % Output input to BT
    u(2) = u_cmd(1);                             % Output input to VSP1
    u(3) = u_cmd(2);                             % Output input to VSP2
    
end

== matlab function Position_Control_PID_CSEI/Heading Controller/MATLAB Function1 ==
  data: psi input; psi_mod output
function psi_mod = wrapToPi(psi)

psi_mod = mod(psi + pi, 2*pi) - pi;

== matlab function Position_Control_PID_CSEI/MATLAB Function3 ==
  data: psi input; psi_mod output
function psi_mod = wrapToPi(psi)

psi_mod = mod(psi + pi, 2*pi) - pi;

== matlab function Position_Control_PID_CSEI/CSEI ==
  data: xdot output; x input; tau input; current input
function xdot  = CSEI(x, tau, current)
%% nu = [u, v, r], eta = [x, y, psi]
%  u:     surge velocity          (m/s)
%  v:     sway velocity           (m/s)
%  r:     yaw velocity            (rad/s)
%  x:     position in x direction (m)
%  y:     position in y direction (m)
%  psi:   yaw angle               (rad)

% This block calculates the change in position and heading given the
% current position and heading and velocities.


% State and current variables
nu = x(1:3); eta = x(4:6);
%% Initializing parameters
R = [cos(eta(3)) -sin(eta(3)) 0;
     sin(eta(3)) cos(eta(3)) 0;
     0 0 1];                        % Rotation matrix with heading
nu_c = R'*[current;0];              % Current velocity vector in body frame
nu_r = nu-nu_c;                     % Relative velocity
u   = nu_r(1);                      % Speed in x
v   = nu_r(2);                      % Speed in y
r   = nu_r(3);                      % Yaw rate

tau = [tau(1);tau(2);tau(3)];
%% MATRICES 
m    = 14.11;   I_z  =  1.7600;   x_g = 0.0375;

%% Added mass
X_ud  =     -2.0;											
					Y_vd =      -10.0;	N_vd =    -0.0;		
					Y_rd =      -0.0;	N_rd =    -1.0;	

%% Total mass matrix
m_11 = m-X_ud;
m_22 = m-Y_vd;
m_23 = m*x_g-Y_rd;
m_32 = m*x_g-N_vd;
m_33 = I_z-N_rd;

M    = [m_11 0    0
        0    m_22 m_23
        0    m_32 m_33];
	
%% Damping coefficients
% Comments at the end of the lines indicate the old values used.
X_u		= -0.6555;		X_v		= 0;
X_uu 	= 0.3545;		X_vv	= -2.443;
X_uuu 	= -3.787;		X_vvv	= 0;

						Y_v		= -1.33; 			Y_r		= -7.250; 
						Y_vv	= -2.776;			Y_rr	= -3.450; 
						Y_vvv	= -64.91;			Y_rrr	= 0;
						
						Y_rv	= -0.805;			Y_vr	= -0.845;

						N_v		= 0;				N_r		= -1.900;
						N_vv	= -0.2088;			N_rr	= -0.750;
						N_vvv	= 0;				N_rrr	= 0;
						
						N_rv	= 0.130;			N_vr	= 0.080;

%% Correolis matrix
c_13 = -(m-Y_vd)*v-(m*x_g-Y_rd)*r;
c_23 = (m-X_ud)*u;
C    = [0     0     c_13
        0     0     c_23
        -c_13 -c_23 0   ];

%% Assembly of the damping matrix
d_11 = -X_u - X_uu*u - X_uuu*u^2;
d_22 = -Y_v - Y_vv*v - Y_vvv*v^2 - Y_rv*abs(r);
d_33 = -N_r - N_rr*abs(r) - N_rrr*r^2 - N_vr*abs(v);

d_12 = -X_v - X_vv*v - X_vvv*v^2;
d_23 = -Y_r - Y_rr*abs(r) - Y_rrr*r^2 - Y_vr*abs(v);
d_32 = -N_v - N_vv*v - N_vvv*v^2 - N_rv*abs(r);

D    = [d_11 0 0
        0    d_22 d_23
        0    d_32 d_33];

%% Initializing
psi = eta(3);                       % Heading
R = [cos(psi) -sin(psi) 0
     sin(psi) cos(psi)  0
     0        0         1];         % Rotation matrix with heading
 
%% Calculating
eta_dot = R*(nu);
%% CALCULATION
nu_dot = M\(tau-(C+D)*nu_r);
% tau_curr = (C+D)*nu_c;
xdot = [nu_dot;  % u, v, r
        eta_dot]; % x, y, psi
end

== matlab function Position_Control_PID_CSEI/MATLAB Function1 ==
  data: psi input; psi_mod output
function psi_mod = wrapToPi(psi)

psi_mod = mod(psi + pi, 2*pi) - pi;

== matlab function Position_Control_PID_CSEI/Thruster modeling/MATLAB Function ==
  data: x1 output size=1; y1 output size=1; u_1 input size=1; a_1 input size=1; moment1 output size=1; f_VSP1_max input
function [x1,y1,moment1] = fcn(u_1, a_1, f_VSP1_max)
% This function takes in the input to VSP1 and calculates the resulting
% forces and moment.
ly_VSP = 0.055;                         % Moment arm along y
lx_VSP = 0.4574;                        % Moment arm along x
% f_VSP1_max = 2.5;                      % Max thrust available

x1 = u_1*f_VSP1_max*cos(a_1);               % Resulting forces in x
y1 = u_1*f_VSP1_max*sin(a_1);               % Resulting forces in y
moment1 = x1*ly_VSP*(1) + y1*lx_VSP*(-1);   % Resulting moment

== matlab function Position_Control_PID_CSEI/MATLAB Function ==
  data: uu input
  
function USV_display(uu)
    x = uu(1);
    y = uu(2);
    psi = uu(3);
    time = uu(4);

    margin = 5; % 시야 여유 공간

    % 선박 외형 정의 (북쪽을 향하도록 설정)
    scale_factor = 0.5;   
    % 기존 선박 모양을 -90도 회전시켜 북쪽(x축) 향하도록 수정
    original_shape_x = [-1 -1 0 1 1 -1];
    original_shape_y = [-1 1 2 1 -1 -1];
    R_init = [cosd(-90), -sind(-90); 
              sind(-90),  cosd(-90)];
    rotated_shape = R_init * [original_shape_x; original_shape_y];
    base_shape_x = rotated_shape(1, :) * scale_factor;
    base_shape_y = rotated_shape(2, :) * scale_factor;

    persistent ship_outline current_position_marker    
    
    if isempty(ship_outline)
        figure(1)
        subplot(121)
        hold on
        scatter(y,x,"blue", "."	);
        axis equal
        xlabel('y (m)');
        ylabel('x (m)'); grid on;

        subplot(122)
        hold on;
        scatter(y,x,"blue", "."	);
        ship_outline = plot(base_shape_x, base_shape_y, 'm-', 'LineWidth', 2); % 초기 선박 외곽선
        current_position_marker = plot(nan, nan, 'ko', 'MarkerSize', 5, 'MarkerFaceColor', 'k'); % 현재 위치       
        axis equal
        xlabel('y (m)');
        ylabel('x (m)'); grid on;
        xlim([x - margin, x + margin]);
        ylim([y - margin, y + margin]);
    end
        subplot(121)
        scatter(y,x,"blue", ".");
        R = [cos(psi), -sin(psi); 
             sin(psi),  cos(psi)];
        rotated_coords = R * [base_shape_x; base_shape_y];
        translated_x = rotated_coords(1, :) + x; % North
        translated_y = rotated_coords(2, :) + y; % East

        subplot(122)
        set(ship_outline, 'XData', translated_y, 'YData', translated_x);
        set(current_position_marker, 'XData', y, 'YData', x);
        scatter(y,x,"blue", "."	);
        xlim([y - margin, y + margin]);
        ylim([x - margin, x + margin]);
        drawnow

end

== matlab function Position_Control_PID_CSEI/Thruster modeling/MATLAB Function1 ==
  data: x2 output size=1; u_2 input size=1; y2 output size=1; a_2 input size=1; moment2 output size=1; f_VSP2_max input
function [x2,y2,moment2] = fcn(u_2,a_2, f_VSP2_max)
% This function takes in the input to VSP2 and calculates the resulting
% forces and moment.
ly_VSP = 0.055;                         % Moment arm along y
lx_VSP = 0.4574;                        % Moment arm along x
% f_VSP2_max = 2.5;                      % Max thrust available

x2 = u_2*f_VSP2_max*cos(a_2);               % Resulting forces in x
y2 = u_2*f_VSP2_max*sin(a_2);               % Resulting forces in y
moment2 = x2*ly_VSP*(-1) + y2*lx_VSP*(-1);  % Resulting moment

== matlab function Position_Control_PID_CSEI/Thruster modeling/MATLAB Function2 ==
  data: u_bt input size=1; y3 output size=1; moment3 output size=1; f_BT_max input
function [y3,moment3] = fcn(u_bt, f_BT_max)
% This function takes in the input to the BT and calculates the resulting
% forces and moment.
lx_BT = 0.3875;         % Moment arm along x
% f_BT_max = 2;         % Max thrust available
    
y3 = u_bt*f_BT_max;     % Resulting force in y
moment3 = y3*lx_BT;     % Resulting moment
